simulink model "HexC_HierarchicalController"  (R2022b)
settings: Solver=VariableStepAuto  StartTime=0.0  StopTime=tot_time  FixedStep=1e-2  RelTol=1e-3
InitFcn:
  | %%% INITIALIZATION
  | 
  | %% CONTROL PARAMETERS
  | 
  | A = [zeros(3, 3), eye(3); zeros(3, 6)];
  | 
  | B = [zeros(3, 3); eye(3)];
  | 
  | p = [-2 -2*10 -2*11 -2*12 -2*13 -2*14];
  | 
  | Kp = place(A, B, p);
  | 
  | p = [-20 -20*10 -20*11 -20*12 -20*13 -20*14];
  | 
  | Ke = place(A, B, p);
  | 
  | Ki = 250*eye(3);
  | Ki_ang = 5000*eye(3);
  | 
  | %% UAV PARAMETERS
  | 
  | mass = 1.56779;
  | Ib = diag([0.0347563, 0.0458929, 0.0977]);
  | 
  | %% ESTIMATOR PARAMETERS
  | 
  | syms s;
  | c_0 = 100;
  | poly = (s + c_0)^3;
  | K_est = double(coeffs(poly));
  | 
  | %% PLANNER (ASSUMING THE POINTS IN path HAVE ALREADY BEEN GENERATED WITH RRT)
  | 
  | Ts = 1e-3;
  | npoints = length(path(:, 1));
  | tseg = 5;
  | ttot=(npoints-1)*tseg; %duration
  | tdead=20; %dead time to evaluate the steady-state
  | tot_time = ttot + tdead;
  | 
  | t1=linspace(0,tseg,round(tseg/Ts));
  | t=linspace(0,ttot+tdead,round(ttot/Ts)+round(tdead/Ts));
  | 
  | psi_0 = deg2rad(0);
  | delta_psi = deg2rad(5);
  | 
  | p_d = []; dot_p_d = []; ddot_p_d = [];
  | 
  | for i = 1:npoints-1
  |     pi= zeros(4,length(t1)); dot_pi= zeros(4,length(t1)); ddot_pi= zeros(4,length(t1));
  |     %Initial and final conditions
  |     x0= path(i, 1); xf=path(i+1, 1); dot_x0= 0; dot_xf=0; ddot_x0=0; ddot_xf=0; dddot_x0 = 0; dddot_xf = 0;
  |     y0= path(i, 2); yf=path(i+1, 2); dot_y0= 0; dot_yf=0; ddot_y0=0; ddot_yf=0; dddot_y0 = 0; dddot_yf = 0;
  |     z0= path(i, 3); zf=path(i+1, 3); dot_z0= 0; dot_zf=0; ddot_z0=0; ddot_zf=0; dddot_z0 = 0; dddot_zf = 0;
  |     psi0 = psi_0+(i-1)*delta_psi;
  |     psif=psi_0+i*delta_psi; dot_psi0= 0; dot_psif=0; ddot_psi0=0; ddot_psif=0; dddot_psi0 = 0; dddot_psif = 0;
  |     p0=[x0,y0,z0,psi0]; dot_p0=[dot_x0,dot_y0,dot_z0,dot_psi0]; ddot_p0=[ddot_x0,ddot_y0,ddot_z0,ddot_psi0]; dddot_p0=[dddot_x0,dddot_y0,dddot_z0,dddot_psi0];
  |     pf=[xf,yf,zf,psif]; dot_pf=[dot_xf,dot_yf,dot_zf,dot_psif]; ddot_pf=[ddot_xf,ddot_yf,ddot_zf,ddot_psif]; dddot_pf=[dddot_xf,dddot_yf,dddot_zf,dddot_psif];
  |     %5-th order polynomial
  |     a0=zeros(1,4); a1=zeros(1,4); a2=zeros(1,4); a3=zeros(1,4); a4=zeros(1,4); a5=zeros(1,4); a6 = zeros(1,4); a7 = zeros(1,4);
  | 
  |     t_iniz = 0;
  |     t_fin = tseg;
  | 
  |     for j=1:4
  |         A = [t_iniz^7, t_iniz^6, t_iniz^5, t_iniz^4, t_iniz^3, t_iniz^2, t_iniz, 1;
  |             t_fin^7, t_fin^6, t_fin^5, t_fin^4, t_fin^3, t_fin^2, t_fin, 1;
  |             7*t_iniz^6, 6*t_iniz^5, 5*t_iniz^4, 4*t_iniz^3, 3*t_iniz^2, 2*t_iniz, 1, 0;
  |             7*t_fin^6, 6*t_fin^5, 5*t_fin^4, 4*t_fin^3, 3*t_fin^2, 2*t_fin, 1, 0;
  |             42*t_iniz^5, 30*t_iniz^4, 20*t_iniz^3, 12*t_iniz^2, 6*t_iniz, 2, 0, 0;
  |             42*t_fin^5, 30*t_fin^4, 20*t_fin^3, 12*t_fin^2, 6*t_fin, 2, 0, 0;
  |             210*t_iniz^4, 120*t_iniz^3, 60*t_iniz^2, 24*t_iniz, 6, 0, 0, 0;
  |             210*t_fin^4, 120*t_fin^3, 60*t_fin^2, 24*t_fin, 6, 0, 0, 0];
  |         b = [p0(j) pf(j) dot_p0(j) dot_pf(j) ddot_p0(j) ddot_pf(j) dddot_p0(j) dddot_pf(j)]';
  |         a_temp = A\b;
  |         a7(j) = a_temp(1);
  |         a6(j) = a_temp(2);
  |         a5(j) = a_temp(3);
  |         a4(j) = a_temp(4);
  |         a3(j) = a_temp(5);
  |         a2(j) = a_temp(6);
  |         a1(j) = a_temp(7);
  |         a0(j) = a_temp(8);
  | 
  |         %trajectories
  |         pi(j,:)=a7(j)*t1.^7 + a6(j)*t1.^6 + a5(j)*t1.^5 +a4(j)*t1.^4 +a3(j)*t1.^3 +a2(j)*t1.^2 +a1(j)*(t1-(i-1)*tseg) +a0(j);
  |         dot_pi(j,:) = 7*a7(j)*t1.^6 + 6*a6(j)*t1.^5 + 5*a5(j)*t1.^4 +4*a4(j)*t1.^3 +3*a3(j)*t1.^2 +2*a2(j)*(t1-(i-1)*tseg) +a1(j);
  |         ddot_pi(j,:) = 42*a7(j)*t1.^5 + 30*a6(j)*t1.^4 + 5*4*a5(j)*t1.^3 +4*3*a4(j)*t1.^2 +3*2*a3(j)*(t1-(i-1)*tseg) +2*a2(j);
  |     end
  | 
  |     p_d = [p_d pi];
  |     dot_p_d = [dot_p_d dot_pi];
  |     ddot_p_d = [ddot_p_d ddot_pi];
  | 
  | end
  | 
  | %addition of the stead-state terms
  | p_d=[p_d zeros(1,round(tdead/Ts))+p_d(:, end)];
  | dot_p_d=[dot_p_d zeros(1,round(tdead/Ts))+dot_p_d(:, end)];
  | ddot_p_d=[ddot_p_d zeros(1,round(tdead/Ts))+ddot_p_d(:, end)];
  | %data for Simulink
  | pos_0 = [x0 y0 z0];
  | lin_vel_0 = [dot_x0 dot_y0 dot_z0];
  | w_bb_0 = [0 0 0];
  | csi_d=p_d(1:3,:); dot_csi_d=dot_p_d(1:3,:); ddot_csi_d=ddot_p_d(1:3,:);
  | psi_d=p_d(4,:); dot_psi_d=dot_p_d(4,:); ddot_psi_d=ddot_p_d(4,:);
  | 
  | %% VISUALIZATION
  | 
  | scene = uavScenario("UpdateRate",100,"StopTime",100,"ReferenceLocation",[0, 0, 0]);
  | scene.addInertialFrame("NED","MAP",trvec2tform([1 0 0]));
  | scene.addMesh("Polygon", {[0 0; 0 20; 20 20; 20 0],[-1 0]},[0.3 0.3 0.3]);
  | scene.addMesh("Polygon", {[0 9; 0 11; 20 11; 20 9],[0 2]},[0 1 1]);
  | scene.addMesh("Polygon", {[0 9; 0 11; 20 11; 20 9],[8 10]},[0 1 1]);
  | scene.addMesh("Polygon", {[0 9; 0 11; 7 11; 7 9],[2 8]},[0 1 1]);
  | scene.addMesh("Polygon", {[20 9; 20 11; 14 11; 14 9],[2 8]},[0 1 1]);
  | scene.addMesh("Polygon", {[1 2; 1 7; 3 7; 3 2],[0 5]},[0 0 1]);
  | scene.addMesh("Cylinder", {[10 5 1],[0 10]}, [0 1 0]);
  | 
  | traj = waypointTrajectory("Waypoints", [0 0 0; 0 0 0; 0 0 0],"TimeOfArrival",[0 1 2]);
  | uavPlat = uavPlatform("UAV",scene,"Trajectory",traj);
  | updateMesh(uavPlat,"quadrotor",{1.5},[1 0 0],[0 0 0],eul2quat([0 0 0]));
values from neighbouring files (symbols this model uses):
  i = i+1    (= 1)    [PlannerRRT.m]
  j = j+meshres    (= 0.1)    [PlannerRRT.m]
  path = [path; roadmap(connections(indexPath-2, 2), :)]    [PlannerRRT.m]
undefined symbols (not defined in the file or in its folder): DiscIntNeverNeededParam
libraries: uavsimlib x3, robotcorelib x1
settings Model: Creator=Federico  LastModifiedBy=Federico
settings OptimizationCC: ZeroExternalMemoryAtStartup=off  ZeroInternalMemoryAtStartup=off
settings RTWCC: GenCodeOnly=on  TargetLang=C++
settings GRTTargetCC: TargetLangStandard=C++11 (ISO)  CodeInterfacePackaging=C++ class

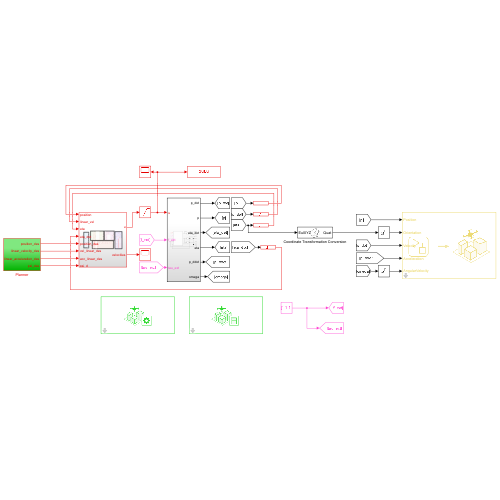
[thumbnail: Simulink's stored preview of the top-level diagram]
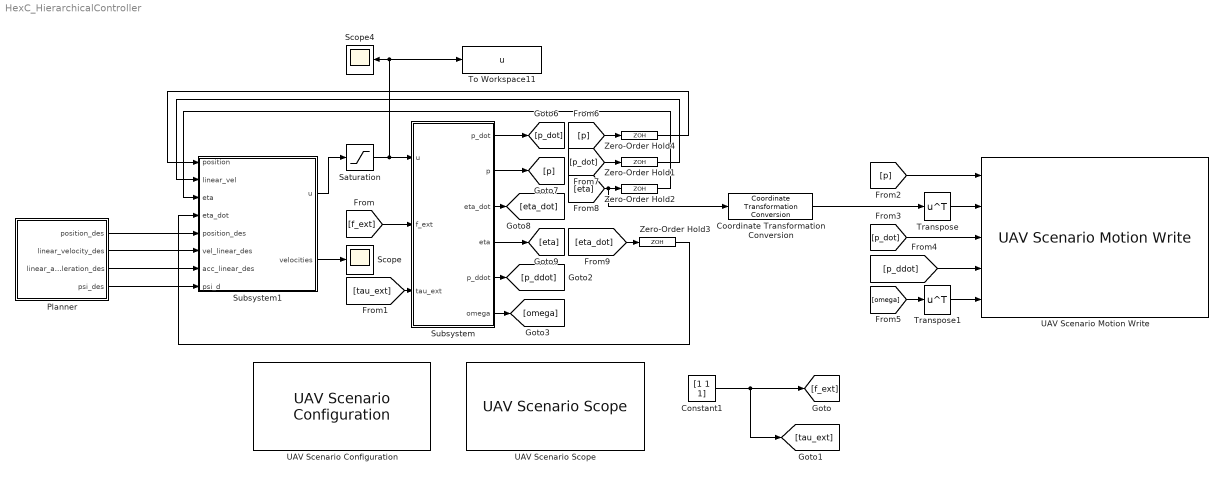
== system HexC_HierarchicalController ==
  Constant1 : Constant  Value=[1 1 1]
  Coordinate Transformation Conversion : robotcorelib/Coordinate Transformation Conversion  InputRepresentation=Euler Angles  InputEulerSequence=XYZ  ShowTrVecInputPort=on  OutputRepresentation=Quaternion  OutputEulerSequence=ZYX  ShowTrVecOutputPort=on  SimulateUsing=Interpreted execution
  Planner : Subsystem
  Saturation : Saturate  UpperLimit=[50 50 50 50 50 50]  LowerLimit=[-50 -50 -50 -50 -50 -50]
  Scope : Scope
  Scope4 : Scope
  Subsystem : Subsystem
  Subsystem1 : Subsystem
  To Workspace11 : ToWorkspace  VariableName=u  SaveFormat=Structure With Time  SampleTime=-1
  Transpose : Math  Operator=transpose
  Transpose1 : Math  Operator=transpose
  UAV Scenario Configuration : uavsimlib/UAV Scenario Configuration  Priority=-1  UAVScenarioObject=scene  SampleTime=0.1  UpdateParam=false  SensorMotionBusName='SensorMotionBus'  PlatformMotionBusName='PlatformMotionBus'  ScenarioMotionBusName='ScenarioMotionBus'  ScenarioMotionSignalName='ScenarioMotions'
  UAV Scenario Motion Write : uavsimlib/UAV Scenario Motion Write  Priority=0  PlatName='UAV'  ReferenceFrame=NED
  UAV Scenario Scope : uavsimlib/UAV Scenario Scope  Priority=1  SensorNameTable={}  SampleTime=0.1
  Zero-Order Hold{1..4} (4 alike) : ZeroOrderHold  SampleTime=Ts
  wires:
  Subsystem/4(eta) -> [eta]
  Subsystem/3(eta_dot) -> [eta_dot]
  [p] -> Zero-Order Hold4/1
  Subsystem/1(p_dot) -> [p_dot]
  [p_dot] -> Zero-Order Hold1/1
  Zero-Order Hold4/1 -> Subsystem1/1(position)
  [eta] -> Coordinate Transformation Conversion/1, Zero-Order Hold2/1
  Subsystem/2(p) -> [p]
  Zero-Order Hold1/1 -> Subsystem1/2(linear_vel)
  Planner/1(position_des) -> Subsystem1/5(position_des)
  Zero-Order Hold2/1 -> Subsystem1/3(eta)
  Planner/2(linear_velocity_des) -> Subsystem1/6(vel_linear_des)
  Planner/3(linear_acceleration_des) -> Subsystem1/7(acc_linear_des)
  Planner/4(psi_des) -> Subsystem1/8(psi_d)
  Subsystem1/1(u) -> Saturation/1
  [eta_dot] -> Zero-Order Hold3/1
  Zero-Order Hold3/1 -> Subsystem1/4(eta_dot)
  [f_ext] -> Subsystem/2(f_ext)
  [tau_ext] -> Subsystem/3(tau_ext)
  Transpose1/1 -> UAV Scenario Motion Write/5
  [p_ddot] -> UAV Scenario Motion Write/4
  [p] -> UAV Scenario Motion Write/1
  [p_dot] -> UAV Scenario Motion Write/3
  [omega] -> Transpose1/1
  Transpose/1 -> UAV Scenario Motion Write/2
  Coordinate Transformation Conversion/1 -> Transpose/1
  Subsystem/5(p_ddot) -> [p_ddot]
  Subsystem/6(omega) -> [omega]
  Subsystem1/2(velocities) -> Scope/1
  Constant1/1 -> [f_ext], [tau_ext]
  Saturation/1 -> To Workspace11/1, Scope4/1, Subsystem/1(u)

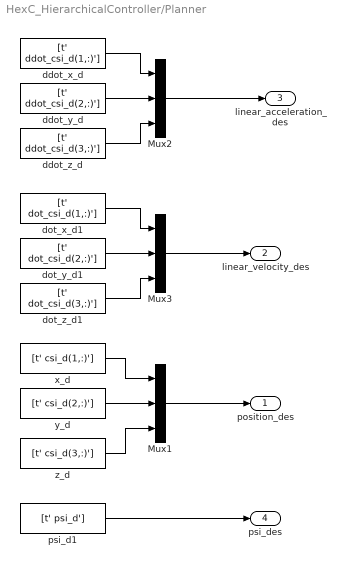
== system HexC_HierarchicalController/Planner ==
  Mux1 : Mux  Inputs=3
  Mux2 : Mux  Inputs=3
  Mux3 : Mux  Inputs=3
  ddot_x_d : FromWorkspace  VariableName=[t' ddot_csi_d(1,:)']  SampleTime=Ts
  ddot_y_d : FromWorkspace  VariableName=[t' ddot_csi_d(2,:)']  SampleTime=Ts
  ddot_z_d : FromWorkspace  VariableName=[t' ddot_csi_d(3,:)']  SampleTime=Ts
  dot_x_d1 : FromWorkspace  VariableName=[t' dot_csi_d(1,:)']  SampleTime=Ts
  dot_y_d1 : FromWorkspace  VariableName=[t' dot_csi_d(2,:)']  SampleTime=Ts
  dot_z_d1 : FromWorkspace  VariableName=[t' dot_csi_d(3,:)']  SampleTime=Ts
  psi_d1 : FromWorkspace  VariableName=[t' psi_d']  SampleTime=Ts
  x_d : FromWorkspace  VariableName=[t' csi_d(1,:)']  SampleTime=Ts
  y_d : FromWorkspace  VariableName=[t' csi_d(2,:)']  SampleTime=Ts
  z_d : FromWorkspace  VariableName=[t' csi_d(3,:)']  SampleTime=Ts
  position_des : Outport
  linear_velocity_des : Outport  Port=2
  linear_acceleration_des : Outport  Port=3
  psi_des : Outport  Port=4
  wires:
  y_d/1 -> Mux1/2
  z_d/1 -> Mux1/3
  x_d/1 -> Mux1/1
  ddot_y_d/1 -> Mux2/2
  ddot_z_d/1 -> Mux2/3
  ddot_x_d/1 -> Mux2/1
  Mux2/1 -> linear_acceleration_des/1
  Mux1/1 -> position_des/1
  dot_y_d1/1 -> Mux3/2
  dot_z_d1/1 -> Mux3/3
  dot_x_d1/1 -> Mux3/1
  Mux3/1 -> linear_velocity_des/1
  psi_d1/1 -> psi_des/1

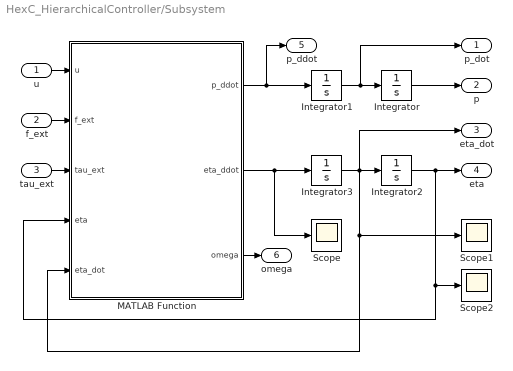
== system HexC_HierarchicalController/Subsystem ==
  u : Inport
  f_ext : Inport  Port=2
  tau_ext : Inport  Port=3
  Integrator : Integrator  InitialCondition=path(1, :)
  Integrator1 : Integrator
  Integrator2 : Integrator  InitialCondition=[0 0 psi_0]
  Integrator3 : Integrator
  MATLAB Function : MATLAB Function  TreatAsAtomicUnit=on
  Scope : Scope
  Scope1 : Scope
  Scope2 : Scope
  p_dot : Outport
  p : Outport  Port=2
  eta_dot : Outport  Port=3
  eta : Outport  Port=4
  p_ddot : Outport  Port=5
  omega : Outport  Port=6
  wires:
  MATLAB Function/1(p_ddot) -> Integrator1/1, p_ddot/1
  Integrator1/1 -> p_dot/1, Integrator/1
  Integrator/1 -> p/1
  u/1 -> MATLAB Function/1(u)
  Integrator3/1 -> MATLAB Function/5(eta_dot), Scope1/1, eta_dot/1, Integrator2/1
  Integrator2/1 -> MATLAB Function/4(eta), Scope2/1, eta/1
  MATLAB Function/2(eta_ddot) -> Scope/1, Integrator3/1
  f_ext/1 -> MATLAB Function/2(f_ext)
  tau_ext/1 -> MATLAB Function/3(tau_ext)
  MATLAB Function/3(omega) -> omega/1

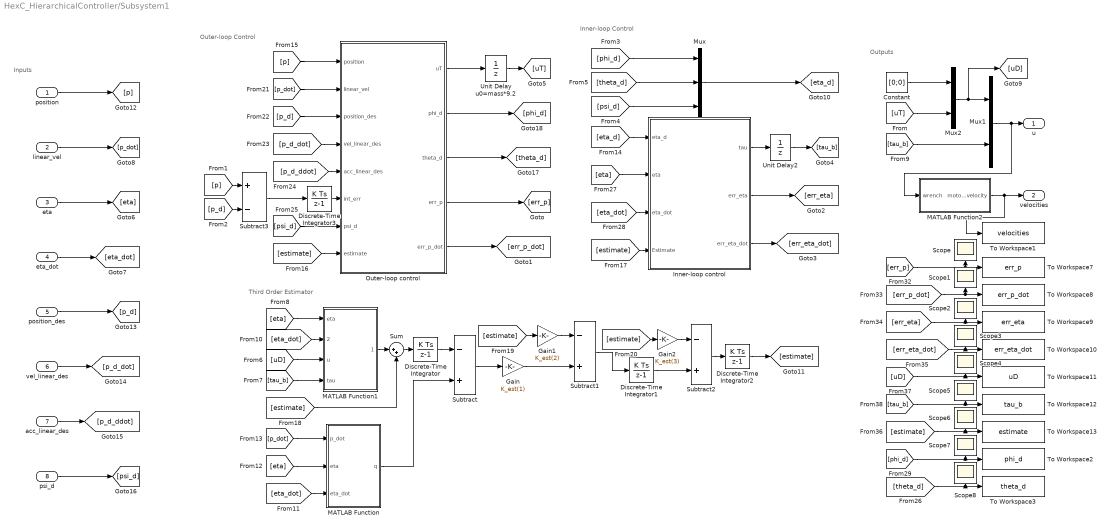
== system HexC_HierarchicalController/Subsystem1 ==
  note: Outputs
  note: Inner-loop Control
  note: Outer-loop Control
  note: Inputs
  note: Third Order Estimator
  position : Inport
  linear_vel : Inport  Port=2
  eta : Inport  Port=3
  eta_dot : Inport  Port=4
  position_des : Inport  Port=5
  vel_linear_des : Inport  Port=6
  acc_linear_des : Inport  Port=7
  psi_d : Inport  Port=8
  Constant : Constant  Value=[0;0]
  Discrete-Time Integrator{,1..3} (4 alike) : DiscreteIntegrator  SampleTime=Ts  ICPrevOutput=DiscIntNeverNeededParam  ICPrevScaledInput=DiscIntNeverNeededParam
  Gain : Gain  Gain=K_est(1)
  Gain1 : Gain  Gain=K_est(2)
  Gain2 : Gain  Gain=K_est(3)
  Inner-loop control : Subsystem
  MATLAB Function : MATLAB Function  TreatAsAtomicUnit=on
  MATLAB Function1 : MATLAB Function  TreatAsAtomicUnit=on
  MATLAB Function2 : MATLAB Function  TreatAsAtomicUnit=on
  Mux : Mux  Inputs=3
  Mux1 : Mux  Inputs=2
  Mux2 : Mux  Inputs=2
  Outer-loop control : MATLAB Function  TreatAsAtomicUnit=on
  Scope{,1..8} (9 alike) : Scope
  Subtract : Sum  Inputs=-+
  Subtract1 : Sum  Inputs=-+
  Subtract2 : Sum  Inputs=-+
  Subtract3 : Sum  Inputs=+-
  Sum : Sum  Inputs=|++
  To Workspace1 : ToWorkspace  VariableName=velocities  SampleTime=-1
  To Workspace10 : ToWorkspace  VariableName=err_eta_dot  SampleTime=-1
  To Workspace11 : ToWorkspace  VariableName=uD  SampleTime=-1
  To Workspace12 : ToWorkspace  VariableName=tau_b  SampleTime=-1
  To Workspace13 : ToWorkspace  VariableName=estimate  SampleTime=-1
  To Workspace2 : ToWorkspace  VariableName=phi_d  SampleTime=-1
  To Workspace3 : ToWorkspace  VariableName=theta_d  SampleTime=-1
  To Workspace7 : ToWorkspace  VariableName=err_p  SampleTime=-1
  To Workspace8 : ToWorkspace  VariableName=err_p_dot  SampleTime=-1
  To Workspace9 : ToWorkspace  VariableName=err_eta  SampleTime=-1
  Unit Delay u0=mass*9.2 : UnitDelay  InitialCondition=mass*9.81  SampleTime=Ts
  Unit Delay2 : UnitDelay  InitialCondition=[0 0 0]  SampleTime=Ts
  u : Outport
  velocities : Outport  Port=2
  wires:
  Inner-loop control/2(err_eta) -> [err_eta]
  Unit Delay2/1 -> [tau_b]
  Outer-loop control/4(err_p) -> [err_p]
  Outer-loop control/5(err_p_dot) -> [err_p_dot]
  Inner-loop control/3(err_eta_dot) -> [err_eta_dot]
  Inner-loop control/1(tau) -> Unit Delay2/1
  eta_dot/1 -> [eta_dot]
  Discrete-Time Integrator2/1 -> [estimate]
  Subtract2/1 -> Discrete-Time Integrator2/1
  [estimate] -> Sum/2
  [uD] -> MATLAB Function1/3(u)
  Subtract1/1 -> Discrete-Time Integrator1/1
  Gain1/1 -> Subtract1/1
  Discrete-Time Integrator1/1 -> Subtract2/2
  [estimate] -> Gain2/1
  Discrete-Time Integrator/1 -> Subtract/1
  Subtract/1 -> Gain/1
  Gain2/1 -> Subtract2/1
  Sum/1 -> Discrete-Time Integrator/1
  [eta_dot] -> MATLAB Function1/2(eta_dot)
  MATLAB Function/1(q) -> Subtract/2
  Gain/1 -> Subtract1/2
  [tau_b] -> MATLAB Function1/4(tau)
  MATLAB Function1/1(model_term) -> Sum/1
  eta/1 -> [eta]
  [p_dot] -> MATLAB Function/1(p_dot)
  linear_vel/1 -> [p_dot]
  [eta] -> MATLAB Function1/1(eta)
  [estimate] -> Gain1/1
  [eta_dot] -> MATLAB Function/3(eta_dot)
  [eta] -> MATLAB Function/2(eta)
  [estimate] -> Outer-loop control/8(estimate)
  [estimate] -> Inner-loop control/4(Estimate)
  position/1 -> [p]
  position_des/1 -> [p_d]
  vel_linear_des/1 -> [p_d_dot]
  acc_linear_des/1 -> [p_d_ddot]
  psi_d/1 -> [psi_d]
  [p] -> Outer-loop control/1(position)
  [p_dot] -> Outer-loop control/2(linear_vel)
  [p_d] -> Outer-loop control/3(position_des)
  [p_d_dot] -> Outer-loop control/4(vel_linear_des)
  [p_d_ddot] -> Outer-loop control/5(acc_linear_des)
  [psi_d] -> Outer-loop control/7(psi_d)
  Outer-loop control/3(theta_d) -> [theta_d]
  Outer-loop control/2(phi_d) -> [phi_d]
  [eta_d] -> Inner-loop control/1(eta_d)
  [eta] -> Inner-loop control/2(eta)
  [eta_dot] -> Inner-loop control/3(eta_dot)
  Mux1/1 -> MATLAB Function2/1(wrench), u/1
  [tau_b] -> Mux1/2
  [err_eta_dot] -> Scope3/1, To Workspace10/1
  [estimate] -> Scope6/1, To Workspace13/1
  [err_eta] -> Scope2/1, To Workspace9/1
  [uD] -> Scope4/1, To Workspace11/1
  [err_p_dot] -> To Workspace8/1, Scope1/1
  [tau_b] -> Scope5/1, To Workspace12/1
  [err_p] -> Scope/1, To Workspace7/1
  Unit Delay u0=mass*9.2/1 -> [uT]
  Mux2/1 -> [uD], Mux1/1
  [uT] -> Mux2/2
  Constant/1 -> Mux2/1
  Outer-loop control/1(uT) -> Unit Delay u0=mass*9.2/1
  [p] -> Subtract3/1
  [p_d] -> Subtract3/2
  Subtract3/1 -> Discrete-Time Integrator3/1
  Discrete-Time Integrator3/1 -> Outer-loop control/6(int_err)
  [theta_d] -> Mux/2
  [psi_d] -> Mux/3
  [phi_d] -> Mux/1
  Mux/1 -> [eta_d]
  MATLAB Function2/1(motor_velocity) -> To Workspace1/1, velocities/1
  [theta_d] -> To Workspace3/1, Scope8/1
  [phi_d] -> To Workspace2/1, Scope7/1

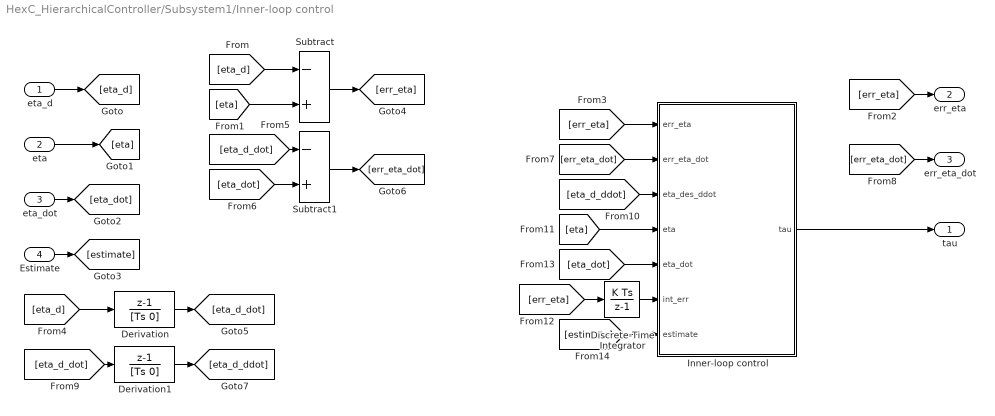
== system HexC_HierarchicalController/Subsystem1/Inner-loop control ==
  eta_d : Inport
  eta : Inport  Port=2
  eta_dot : Inport  Port=3
  Estimate : Inport  Port=4
  Derivation : DiscreteTransferFcn  Numerator=[1 -1]  Denominator=[Ts 0]  SampleTime=Ts
  Derivation1 : DiscreteTransferFcn  Numerator=[1 -1]  Denominator=[Ts 0]  SampleTime=Ts
  Discrete-Time Integrator : DiscreteIntegrator  SampleTime=-1  ICPrevOutput=DiscIntNeverNeededParam  ICPrevScaledInput=DiscIntNeverNeededParam
  Inner-loop control : MATLAB Function  TreatAsAtomicUnit=on
  Subtract : Sum  Inputs=-+
  Subtract1 : Sum  Inputs=-+
  tau : Outport
  err_eta : Outport  Port=2
  err_eta_dot : Outport  Port=3
  wires:
  Inner-loop control/1(tau) -> tau/1
  eta_d/1 -> [eta_d]
  eta/1 -> [eta]
  eta_dot/1 -> [eta_dot]
  Estimate/1 -> [estimate]
  [eta_d] -> Subtract/1
  [eta] -> Subtract/2
  Subtract/1 -> [err_eta]
  [err_eta] -> err_eta/1
  [err_eta] -> Inner-loop control/1(err_eta)
  [eta_d] -> Derivation/1
  Derivation/1 -> [eta_d_dot]
  Subtract1/1 -> [err_eta_dot]
  [eta_dot] -> Subtract1/2
  [eta_d_dot] -> Subtract1/1
  [err_eta_dot] -> Inner-loop control/2(err_eta_dot)
  [err_eta_dot] -> err_eta_dot/1
  [eta_d_dot] -> Derivation1/1
  Derivation1/1 -> [eta_d_ddot]
  [eta_d_ddot] -> Inner-loop control/3(eta_des_ddot)
  [eta] -> Inner-loop control/4(eta)
  Discrete-Time Integrator/1 -> Inner-loop control/6(int_err)
  [err_eta] -> Discrete-Time Integrator/1
  [eta_dot] -> Inner-loop control/5(eta_dot)
  [estimate] -> Inner-loop control/7(estimate)

== matlab function HexC_HierarchicalController/Subsystem1/MATLAB Function2 ==
  data: wrench input; motor_velocity output
function motor_velocity = fcn(wrench)

    z_disp = -0.037;
    l = 0.215;
    b = deg2rad(20);
    
    W_des = [-wrench(1:3); wrench(4:6)];
    gamma = 0.016;
    ct = 8.54858e-6;
    cq = ct*gamma;
    
    xi0 = [l*cosd(-30); l*sind(-30); z_disp];
    xi1 = [l*cosd(-90); l*sind(-90); z_disp];
    xi2 = [l*cosd(-150); l*sind(-150); z_disp];
    xi3 = [l*cosd(150); l*sind(150); z_disp];
    xi4 = [l*cosd(90); l*sind(90); z_disp];
    xi5 = [l*cosd(30); l*sind(30); z_disp];
    
    R0 = Rz(-30)*Rx(-160);
    
    R1 = Rz(-90)*Rx(160);
    
    R2 = Rz(-150)*Rx(-160);
    
    R3 = Rz(150)*Rx(160);
    
    R4 = Rz(90)*Rx(-160);
    
    R5 = Rz(30)*Rx(160);
    
    z = [0;0;1];
    
    M = [-gamma*R0*z+skew(xi0)*R0*z, gamma*R1*z+skew(xi1)*R1*z, -gamma*R2*z+skew(xi2)*R2*z, gamma*R3*z+skew(xi3)*R3*z, -gamma*R4*z+skew(xi4)*R4*z, gamma*R5*z+skew(xi5)*R5*z;
        R0*z, R1*z, R2*z, R3*z, R4*z, R5*z];
    
    M_bar = [M(4:6, :); M(1:3, :)];
    
    lambda = M_bar\W_des;
    omega2 = lambda/ct;
    motor_velocity = sqrt(abs(omega2)).*sign(omega2);

end

function S = skew(v)
    if(numel(v)~= 1)
        S= [0 -v(3) v(2); 
            v(3) 0 -v(1);
            -v(2) v(1) 0];
    else
        S= zeros(3);
    end
end

function S = Rz(a) % In degrees
    S = [cosd(a) -sind(a) 0;
        sind(a) cosd(a) 0;
        0 0 1];
end

function S = Rx(a) % In degrees
    S = [1 0 0;
        0 cosd(a) -sind(a);
        0 sind(a) cosd(a)];
end

== matlab function HexC_HierarchicalController/Subsystem1/MATLAB Function ==
  data: p_dot input size=3; q output size=6; eta input size=3; eta_dot input size=3; mass parameter size=1; Ib parameter size=[3,3]
function q = fcn(p_dot, eta, eta_dot, mass, Ib)

    phi = eta(1);
    theta = eta(2);
    psi = eta(3);
    phi_dot = eta_dot(1);
    theta_dot = eta_dot(2);
    psi_dot = eta_dot(3);
    Q = [1 0         -sin(theta);
         0 cos(phi)  cos(theta)*sin(phi);
         0 -sin(phi) cos(theta)*cos(phi)];
    Q_dot = [0 0                 -theta_dot*cos(theta);
             0 -phi_dot*sin(phi) -theta_dot*sin(theta)*sin(phi)+phi_dot*cos(theta)*cos(phi);
             0 -phi_dot*cos(phi) -theta_dot*sin(theta)*cos(phi)-phi_dot*cos(theta)*sin(phi)];
    M = Q'*Ib*Q;
    C = Q'*skew(Q*eta_dot)*Ib*Q+Q'*Ib*Q_dot;
    
    q = [mass*eye(3) zeros(3, 3);
         zeros(3, 3) M]*[p_dot; eta_dot];
    
end

function S = skew(v)
    if(numel(v)~= 1)
        S= [0 -v(3) v(2); 
            v(3) 0 -v(1);
            -v(2) v(1) 0];
    else
        S= zeros(3);
    end
end

== matlab function HexC_HierarchicalController/Subsystem/MATLAB Function ==
  data: u input size=6; f_ext input; tau_ext input; eta input size=3; eta_dot input size=3; mass parameter size=1; p_ddot output size=3; eta_ddot output size=3; Ib parameter size=[3, 3]; omega output
% UAV model

function [p_ddot, eta_ddot, omega] = fcn(u, f_ext, tau_ext, eta, eta_dot, mass, Ib)

    g = 9.81;

    R = eul2rotm(eta', "XYZ");
    
    f = u(1:3);
    tau = u(4:6); 

    phi = eta(1);
    theta = eta(2);
    psi = eta(3);
    phi_dot = eta_dot(1);
    theta_dot = eta_dot(2);
    psi_dot = eta_dot(3);
    Q = [1 0         -sin(theta);
         0 cos(phi)  cos(theta)*sin(phi);
         0 -sin(phi) cos(theta)*cos(phi)];
    Q_dot = [0 0                 -theta_dot*cos(theta);
             0 -phi_dot*sin(phi) -theta_dot*sin(theta)*sin(phi)+phi_dot*cos(theta)*cos(phi);
             0 -phi_dot*cos(phi) -theta_dot*sin(theta)*cos(phi)-phi_dot*cos(theta)*sin(phi)];
    M = Q'*Ib*Q;
    C = Q'*skew(Q*eta_dot)*Ib*Q+Q'*Ib*Q_dot;


    p_ddot = g*[0;0;1]-1/mass*R*f + f_ext/mass;
    eta_ddot = M\(-C*eta_dot+Q'*tau + tau_ext);
    omega = Q*eta_dot;

end

function S = skew(v)
    if(numel(v)~= 1)
        S= [0 -v(3) v(2); 
            v(3) 0 -v(1);
            -v(2) v(1) 0];
    else
        S= zeros(3);
    end
end

== matlab function HexC_HierarchicalController/Subsystem1/Outer-loop control ==
  data: position input size=3; uT output size=1; linear_vel input size=3; phi_d output size=1; theta_d output size=1; mass parameter size=1; position_des input size=3; vel_linear_des input size=3; acc_linear_des input size=3; int_err input size=3; err_p output size=3; err_p_dot output size=3; psi_d input size=1; Kp parameter size=[3,6]; estimate input size=6; Ki parameter size=[3,3]
function [uT, phi_d, theta_d, err_p, err_p_dot] = fcn(position, ...
    linear_vel, mass, position_des, vel_linear_des, acc_linear_des, ...
    int_err, psi_d, Kp, estimate, Ki)

    g = 9.81;
    
    err_p = position - position_des;
    err_p_dot = linear_vel - vel_linear_des;
    
    mu_d = -Kp*[err_p; err_p_dot]-Ki*int_err+acc_linear_des-1/mass*estimate(1:3);
    
    if (mu_d(3)>g)
        mu_d(3) = 9.8;
    end
    
    uT = mass*sqrt(mu_d(1)^2+mu_d(2)^2+(mu_d(3)-g)^2);
    phi_d = asin(mass/uT*(mu_d(2)*cos(psi_d)-mu_d(1)*sin(psi_d)));
    theta_d = atan((mu_d(1)*cos(psi_d)+mu_d(2)*sin(psi_d))/(mu_d(3)-g));

end

== matlab function HexC_HierarchicalController/Subsystem1/Inner-loop control/Inner-loop control ==
  data: tau output size=3; err_eta input size=3; err_eta_dot input size=3; eta_des_ddot input size=3; eta input; eta_dot input; Ke parameter; int_err input size=3; Ib parameter; estimate input size=6; Ki_ang parameter size=[3,3]
function tau  = fcn(err_eta, err_eta_dot, eta_des_ddot, eta, eta_dot, Ke, ...
    int_err, Ib, estimate, Ki_ang)

    tau_tilde = -Ke*[err_eta; err_eta_dot]-Ki_ang*int_err+eta_des_ddot;
    
    phi = eta(1);
    theta = eta(2);
    psi = eta(3);
    phi_dot = eta_dot(1);
    theta_dot = eta_dot(2);
    psi_dot = eta_dot(3);
    Q = [1 0         -sin(theta);
         0 cos(phi)  cos(theta)*sin(phi);
         0 -sin(phi) cos(theta)*cos(phi)];
    Q_dot = [0 0                 -theta_dot*cos(theta);
             0 -phi_dot*sin(phi) -theta_dot*sin(theta)*sin(phi)+phi_dot*cos(theta)*cos(phi);
             0 -phi_dot*cos(phi) -theta_dot*sin(theta)*cos(phi)-phi_dot*cos(theta)*sin(phi)];
    M = Q'*Ib*Q;
    C = Q'*skew(Q*eta_dot)*Ib*Q+Q'*Ib*Q_dot;
    
    tau = Ib*Q*tau_tilde+inv(Q')*C*eta_dot-Q'*estimate(4:6);

end

function S = skew(v)
    if(numel(v)~= 1)
        S= [0 -v(3) v(2); 
            v(3) 0 -v(1);
            -v(2) v(1) 0];
    else
        S= zeros(3);
    end
end

== matlab function HexC_HierarchicalController/Subsystem1/MATLAB Function1 ==
  data: eta input size=3; eta_dot input size=3; u input size=3; tau input size=3; model_term output size=6; mass parameter size=1; Ib parameter size=[3,3]
function model_term = fcn(eta, eta_dot, u, tau, mass, Ib)

    R = eul2rotm(eta', "XYZ");
    g = 9.81;
    
    phi = eta(1);
    theta = eta(2);
    psi = eta(3);
    phi_dot = eta_dot(1);
    theta_dot = eta_dot(2);
    psi_dot = eta_dot(3);
    Q = [1 0         -sin(theta);
         0 cos(phi)  cos(theta)*sin(phi);
         0 -sin(phi) cos(theta)*cos(phi)];
    Q_dot = [0 0                 -theta_dot*cos(theta);
             0 -phi_dot*sin(phi) -theta_dot*sin(theta)*sin(phi)+phi_dot*cos(theta)*cos(phi);
             0 -phi_dot*cos(phi) -theta_dot*sin(theta)*cos(phi)-phi_dot*cos(theta)*sin(phi)];
    M = Q'*Ib*Q;
    C = Q'*skew(Q*eta_dot)*Ib*Q+Q'*Ib*Q_dot;
    
    model_term = [mass*[0;0;g]-R*u;
        C'*eta_dot+Q'*tau];

end

function S = skew(v)
    if(numel(v)~= 1)
        S= [0 -v(3) v(2); 
            v(3) 0 -v(1);
            -v(2) v(1) 0];
    else
        S= zeros(3);
    end
end
